simulink model "HighwayLaneChangeTestBench"  (R2024b)
settings: Solver=FixedStepAuto  StartTime=0.0  StopTime=scenario.StopTime  FixedStep=Ts  RelTol=1e-3
PostLoadFcn:
  | helperSLHighwayLaneChangeSetup;
values from neighbouring files (symbols this model uses):
  camera = cameraParams(egoActor)    [helperSLHighwayLaneChangeSetup.m]
undefined symbols (not defined in the file or in its folder): actorProfiles, driving, egoFrontExt, egoTTC, enableCCBehavior, enableLCBehavior, enableLCFBehavior, frontSafetyGap, latDevCost, mapInfo, matlabshared, maxAccel, maxCurvature, maxPlanningHorizon, maxYawRate, minVelocity, nextTTC, preferredLane, rearSafetyGap, replanRate, setSpeed, speedCost, targetFrontExt, timeCost, timeHorizon, timeResolution, Ts
libraries: drivingscenarioandsensors x8, canoelib x5, sensorinslib x1
CloseFcn:
  | helperSLHighwayLaneChangeCleanUp;
settings Model: Creator=The MathWorks, Inc.  LastModifiedBy=USER
settings SolverCC: ZeroCrossAlgorithm=Adaptive  AlgebraicLoopSolver=TrustRegion  MaxZcPerStep=1
settings DataIOCC: SaveOutput=off  ReturnWorkspaceOutputs=off
settings OptimizationCC: ReuseModelBlockBuffer=off
settings DebuggingCC: MaskedZcDiagnostic=none  IgnoredZcDiagnostic=none  UnconnectedInputMsg=warning  UnconnectedOutputMsg=warning  UnconnectedLineMsg=warning  BusObjectLabelMismatch=none  SubsystemReferenceDiagnosticForUnitTest=warning
settings ModelReferenceCC: EnableRefExpFcnMdlSchedulingChecks=on
settings RTWCC: GPUComputeCapability=3.5  DLArmComputeVersion=19.05

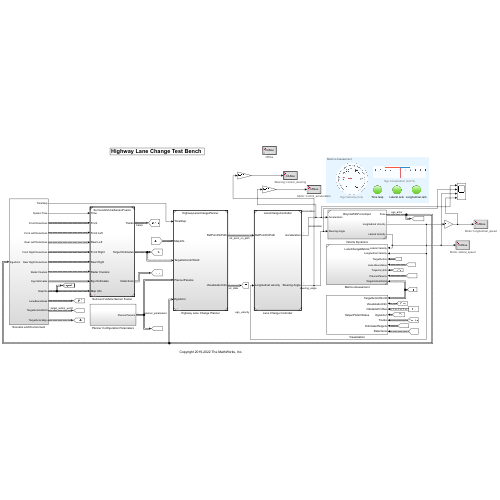
[thumbnail: Simulink's stored preview of the top-level diagram]
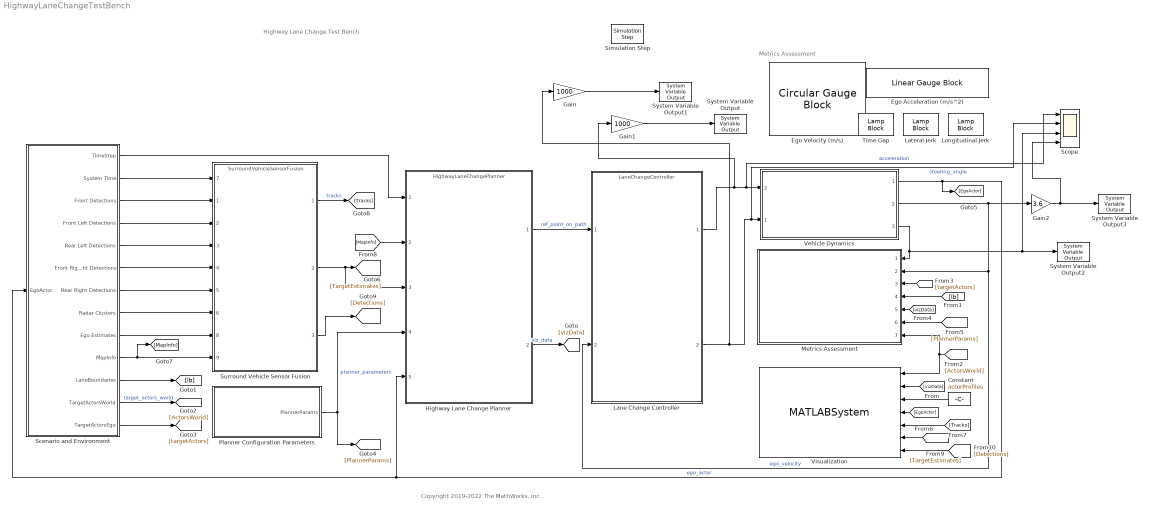
== system HighwayLaneChangeTestBench ==
  note: Copyright 2019-2022 The MathWorks, Inc.
  note: Metrics Assessment
  note: Highway Lane Change Test Bench
  Constant : Constant  Value=actorProfiles  OutDataTypeStr=Bus: BusActorProfiles
  Ego Acceleration (m/s^2) : LinearGaugeBlock  LabelPosition=Hide  ScaleMin=-5  ScaleMax=5
  Ego Velocity (m/s) : CircularGaugeBlock  LabelPosition=Hide  ScaleMax=50  TickInterval=5
  Gain : Gain  Gain=1000
  Gain1 : Gain  Gain=1000
  Gain2 : Gain  Gain=3.6
  Highway Lane Change Planner : ModelReference  ModelNameDialog=HighwayLaneChangePlanner.slx  SimulationMode=Normal  ModelReferenceVersion=10.0
  Lane Change Controller : ModelReference  ModelNameDialog=LaneChangeController.slx  SimulationMode=Normal  ModelReferenceVersion=9.0
  Lateral Jerk : LampBlock  LabelPosition=Hide
  Longitudinal Jerk : LampBlock  LabelPosition=Hide
  Metrics Assessment : Subsystem  ReferencedSubsystem=LaneChangeMetrics
  Planner Configuration Parameters : Subsystem
  Scenario and Environment : Subsystem
  Scope : Scope  NumInputPorts=4
  Simulation Step : canoelib/CANoe I//O/Simulation Step  mode=Offline
      settings: AttributesFormatString=%<mode>  SourceProductName=Vector CANoe
  Surround Vehicle Sensor Fusion : ModelReference  ModelNameDialog=SurroundVehicleSensorFusion.slx  SimulationMode=Normal  ModelReferenceVersion=10.0
      settings: PortSchema="{\"entries\":[{\"content\":{\"sides\":[{\"content\":{\"connectorIds\":[\"In7\",\"In1\",\"In2\",\"In3\",\"In4\",\"In5\",\"In6\",\"In8\",\"In9\"]},\"type\":\"ConnectorPlacement.EquallySpacedRectSide\",\"uuid\":\"babc32b8-473b-4a04-b824-251f7900e603\"},{\"content\":{\"connectorIds\":[\"Out1\",\"Out2\",\"Out3\"],\"side\":\"RIGHT\"},\"type\":\"ConnectorPlacement.EquallySpacedRectSide\",\"uuid\":\"6521796d-8396-47d7-a507-be3f8604ea95\"},{\"content\":{\"connectorIds\":[],\"side\":\"TOP\"},\"type\":\"ConnectorPlacement.EquallySpacedRectSide\",\"uuid\":\"3afcd3a1-01f6-437b-a186-b4f18cfd5e31\"}]},\"type\":\"ConnectorPlacement.EquallySpacedConnector\",\"uuid\":\"2716b65b-56e0-49c3-bc67-2edcf12b2a8e\"}],\"packageUris\":[\"http://schema.mathworks.com/mf0/Connector/R2020b\"],\"version\":\"1.0\"}"
  System Variable Output : canoelib/CANoe I//O/System Variable Output  nsName=Motor  sysVarName=control_acceleration  arrayIndex=-1  rawValue=Default  dataType=Default  dataTypeDB=double  hasEncoding=off  dataTypeCANoe=Get from CANoe
      settings: AttributesFormatString=%<nsName>::%<sysVarName>  SourceProductName=Vector CANoe
  System Variable Output1 : canoelib/CANoe I//O/System Variable Output  nsName=Steering  sysVarName=control_steering  arrayIndex=-1  rawValue=Default  dataType=Default  dataTypeDB=int32  hasEncoding=off  dataTypeCANoe=Get from CANoe
      settings: AttributesFormatString=%<nsName>::%<sysVarName>  SourceProductName=Vector CANoe
  System Variable Output2 : canoelib/CANoe I//O/System Variable Output  nsName=Motor  sysVarName=lateral_speed  arrayIndex=-1  rawValue=Default  dataType=Default  dataTypeDB=int32  hasEncoding=off  dataTypeCANoe=Get from CANoe
      settings: AttributesFormatString=%<nsName>::%<sysVarName>  SourceProductName=Vector CANoe
  System Variable Output3 : canoelib/CANoe I//O/System Variable Output  nsName=Motor  sysVarName=longitudinal_speed  arrayIndex=-1  rawValue=Default  dataType=Default  dataTypeDB=int32  hasEncoding=off  dataTypeCANoe=Get from CANoe
      settings: AttributesFormatString=%<nsName>::%<sysVarName>  SourceProductName=Vector CANoe
  Time Gap : LampBlock  LabelPosition=Hide
  Vehicle Dynamics : Subsystem  ReferencedSubsystem=BicycleWithForceInput
      settings: PortSchema="{\"entries\":[{\"content\":{\"sides\":[{\"content\":{\"connectorIds\":[\"In2\",\"In1\"]},\"type\":\"ConnectorPlacement.EquallySpacedRectSide\",\"uuid\":\"f63f66bc-f59a-4e63-885b-0681004bade6\"},{\"content\":{\"connectorIds\":[\"Out1\",\"Out2\",\"Out3\"],\"side\":\"RIGHT\"},\"type\":\"ConnectorPlacement.EquallySpacedRectSide\",\"uuid\":\"8ac8ea57-0210-4a13-ad95-4f0a9335ab33\"},{\"content\":{\"side\":\"TOP\"},\"type\":\"ConnectorPlacement.EquallySpacedRectSide\",\"uuid\":\"6d0b300d-41b2-47ad-8d2f-35db0d33cdc5\"}]},\"type\":\"ConnectorPlacement.EquallySpacedConnector\",\"uuid\":\"3215dd89-c688-4582-a904-15ea546ef61a\"}],\"packageUris\":[\"http://schema.mathworks.com/mf0/Connector/R2020b\"],\"version\":\"1.0\"}"
  Visualization : MATLABSystem  System=HelperPlotLCStatus  ActorsInfo=Tracks  EnableTopView=on  EnableTrajTopView=on  EnableTracksTopView=on  EnableChaseView=on  EnableTrajChase=on  EnableCaplistChaseView=on  EnableTracksChaseView=on
      mask Type: HelperPlotLCStatus
      mask Display:
      | disp('HelperPlotLCStatus');
      | port_label('input',1,'TargetActorsWorld');
      | port_label('input',2,'VisualizationInfo');
      | port_label('input',3,'ObstacleProfiles');
      | port_label('input',4,'EgoActor');
      | port_label('input',5,'Tracks');
      | port_label('input',6,'EstimatedTargets');
      | port_label('input',7,'Detections');
  wires:
  Planner Configuration Parameters/1(PlannerParams) -> Highway Lane Change Planner/4, [PlannerParams]  "planner_parameters"
  Highway Lane Change Planner/2 -> [vizData]  "viz_data"
  Scenario and Environment/11(LaneBoundaries) -> [lb]
  [lb] -> Metrics Assessment/4
  Highway Lane Change Planner/1 -> Lane Change Controller/1  "ref_point_on_path"
  [ActorsWorld] -> Metrics Assessment/7, Visualization/1
  Scenario and Environment/12(TargetActorsWorld) -> [ActorsWorld]  "target_actors_world"
  Scenario and Environment/13(TargetActorsEgo) -> [targetActors]
  [targetActors] -> Metrics Assessment/3
  Scenario and Environment/1(TimeStep) -> Highway Lane Change Planner/1
  Vehicle Dynamics/1 -> Scenario and Environment/1(EgoActor), Highway Lane Change Planner/5, [EgoActor]  "ego_actor"
  Vehicle Dynamics/2 -> Gain2/1, Lane Change Controller/2, Metrics Assessment/2  "ego_velocity"
  Lane Change Controller/2 -> Gain/1, Scope/2, Vehicle Dynamics/1  "steering_angle"
  Lane Change Controller/1 -> Gain1/1, Scope/1, Vehicle Dynamics/2  "acceleration"
  [vizData] -> Metrics Assessment/5
  [PlannerParams] -> Metrics Assessment/6
  Scenario and Environment/3(Front Detections) -> Surround Vehicle Sensor Fusion/1
  Scenario and Environment/4(Front Left Detections) -> Surround Vehicle Sensor Fusion/2
  Scenario and Environment/5(" Rear Left Detections") -> Surround Vehicle Sensor Fusion/3
  Scenario and Environment/6(Front Right Detections) -> Surround Vehicle Sensor Fusion/4
  Scenario and Environment/7(Rear Right Detections) -> Surround Vehicle Sensor Fusion/5
  Scenario and Environment/8(Radar Clusters) -> Surround Vehicle Sensor Fusion/6
  Scenario and Environment/9(Ego Estimates) -> Surround Vehicle Sensor Fusion/8
  [vizData] -> Visualization/2
  Constant/1 -> Visualization/3
  Scenario and Environment/10(MapInfo) -> [MapInfo], Surround Vehicle Sensor Fusion/9
  [MapInfo] -> Highway Lane Change Planner/2
  Surround Vehicle Sensor Fusion/2 -> Highway Lane Change Planner/3, [TargetEstimates]
  Surround Vehicle Sensor Fusion/1 -> [Tracks]  "tracks"
  Surround Vehicle Sensor Fusion/3 -> [Detections]
  [Tracks] -> Visualization/5
  [Detections] -> Visualization/7
  [EgoActor] -> Visualization/4
  [TargetEstimates] -> Visualization/6
  Scenario and Environment/2(System Time) -> Surround Vehicle Sensor Fusion/7
  Vehicle Dynamics/3 -> Metrics Assessment/1, System Variable Output2/1, Scope/3
  Gain/1 -> System Variable Output1/1
  Gain1/1 -> System Variable Output/1
  Gain2/1 -> Scope/4, System Variable Output3/1

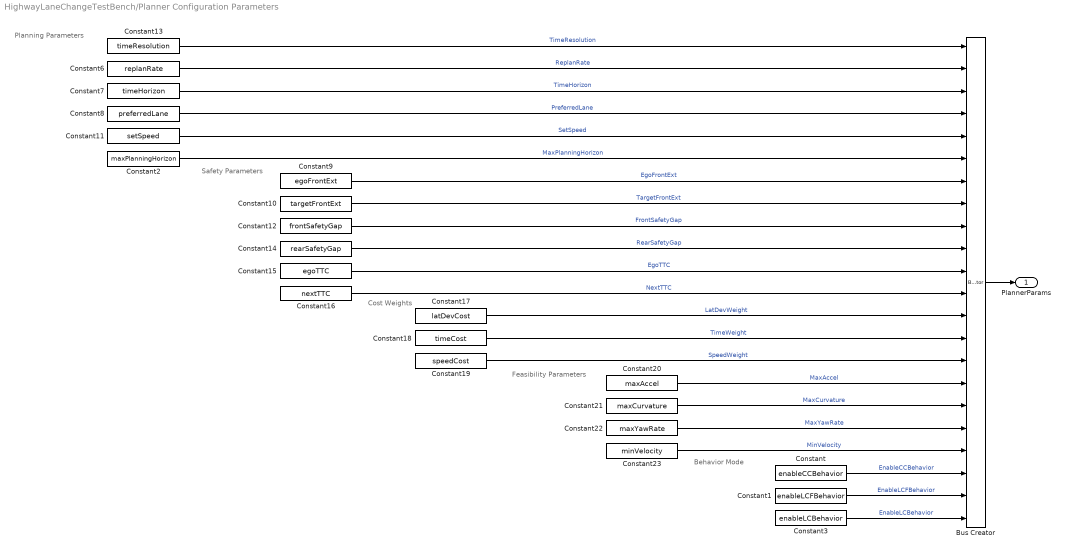
== system HighwayLaneChangeTestBench/Planner Configuration Parameters ==
  note: Planning Parameters
  note: Safety Parameters
  note: Cost Weights
  note: Feasibility Parameters
  note: Behavior Mode
  Bus Creator : BusCreator  Inputs=22  OutDataTypeStr=Bus: BusPlannerParams  NonVirtualBus=on
  Constant : Constant  Value=enableCCBehavior
  Constant1 : Constant  Value=enableLCFBehavior
  Constant10 : Constant  Value=targetFrontExt
  Constant11 : Constant  Value=setSpeed
  Constant12 : Constant  Value=frontSafetyGap
  Constant13 : Constant  Value=timeResolution
  Constant14 : Constant  Value=rearSafetyGap
  Constant15 : Constant  Value=egoTTC
  Constant16 : Constant  Value=nextTTC
  Constant17 : Constant  Value=latDevCost
  Constant18 : Constant  Value=timeCost
  Constant19 : Constant  Value=speedCost
  Constant2 : Constant  Value=maxPlanningHorizon
  Constant20 : Constant  Value=maxAccel
  Constant21 : Constant  Value=maxCurvature
  Constant22 : Constant  Value=maxYawRate
  Constant23 : Constant  Value=minVelocity
  Constant3 : Constant  Value=enableLCBehavior
  Constant6 : Constant  Value=replanRate
  Constant7 : Constant  Value=timeHorizon
  Constant8 : Constant  Value=preferredLane
  Constant9 : Constant  Value=egoFrontExt
  PlannerParams : Outport  OutDataTypeStr=Bus: BusPlannerParams
  wires:
  Constant19/1 -> Bus Creator/15  "SpeedWeight"
  Constant15/1 -> Bus Creator/11  "EgoTTC"
  Constant12/1 -> Bus Creator/9  "FrontSafetyGap"
  Constant6/1 -> Bus Creator/2  "ReplanRate"
  Constant14/1 -> Bus Creator/10  "RearSafetyGap"
  Constant20/1 -> Bus Creator/16  "MaxAccel"
  Constant18/1 -> Bus Creator/14  "TimeWeight"
  Constant11/1 -> Bus Creator/5  "SetSpeed"
  Constant13/1 -> Bus Creator/1  "TimeResolution"
  Constant23/1 -> Bus Creator/19  "MinVelocity"
  Constant9/1 -> Bus Creator/7  "EgoFrontExt"
  Constant16/1 -> Bus Creator/12  "NextTTC"
  Constant10/1 -> Bus Creator/8  "TargetFrontExt"
  Constant7/1 -> Bus Creator/3  "TimeHorizon"
  Constant21/1 -> Bus Creator/17  "MaxCurvature"
  Constant8/1 -> Bus Creator/4  "PreferredLane"
  Constant17/1 -> Bus Creator/13  "LatDevWeight"
  Bus Creator/1 -> PlannerParams/1
  Constant22/1 -> Bus Creator/18  "MaxYawRate"
  Constant/1 -> Bus Creator/20  "EnableCCBehavior"
  Constant1/1 -> Bus Creator/21  "EnableLCFBehavior"
  Constant3/1 -> Bus Creator/22  "EnableLCBehavior"
  Constant2/1 -> Bus Creator/6  "MaxPlanningHorizon"

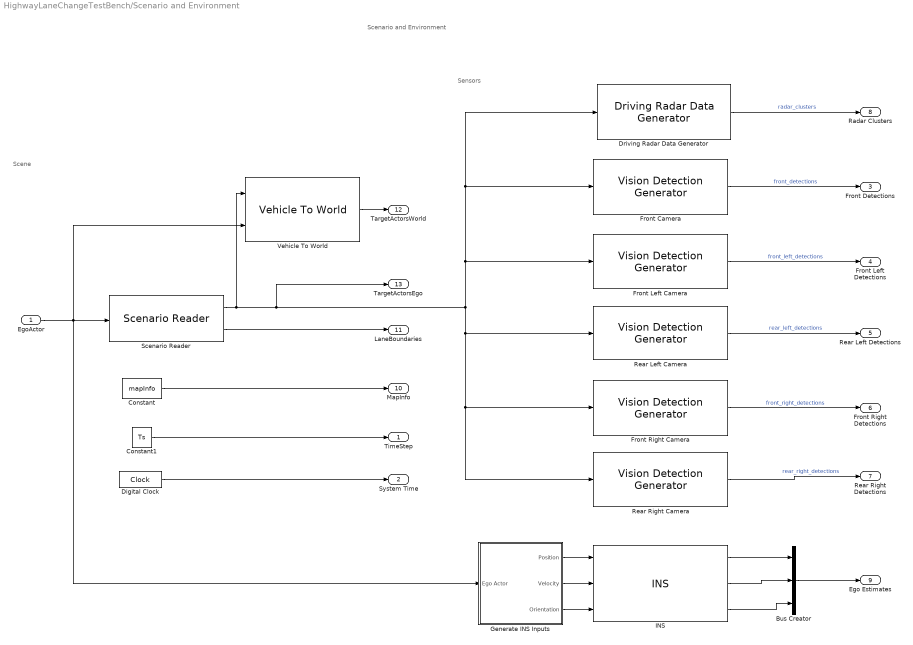
== system HighwayLaneChangeTestBench/Scenario and Environment ==
  note: Sensors
  note: Scene
  note: Scenario and Environment
  EgoActor : Inport
  Bus Creator : BusCreator  Inputs=3
  Constant : Constant  Value=mapInfo  OutDataTypeStr=Bus: BusMapInfo
  Constant1 : Constant  Value=Ts
  Digital Clock : DigitalClock  SampleTime=Ts
  Driving Radar Data Generator : drivingscenarioandsensors/Driving Radar Data Generator  SensorIndex=1  UpdateRate=10  MountingLocation=radar.Position  MountingAngles=radar.Rotation  HasElevation=off  HasRangeRate=on  HasNoise=on  HasFalseAlarms=off  HasOcclusion=off  MaxNumReportsSource=Property  MaxNumReports=50  TargetReportFormat=Clustered detections  DetectionCoordinates=Sensor spherical  TrackCoordinates=Body  BusNameSource=Property  BusName=BusDrivingRadarDataGenerator  SimulateUsing=Interpreted execution  AzimuthResolution=4  ElevationResolution=5  RangeResolution=2.5  RangeRateResolution=0.5  AzimuthBiasFraction=0.1  ElevationBiasFraction=0.1  RangeBiasFraction=0.05  RangeRateBiasFraction=0.05  FieldOfView=radar.FieldOfView  RangeLimits=radar.DetectionRanges  RangeRateLimits=[ -100, 100 ]  DetectionProbability=1  FalseAlarmRate=1e-06  ReferenceRange=100  ReferenceRCS=10  CenterFrequency=77e9  FilterInitializationFcn=initcvekf  ConfirmationThreshold=[2 3]  DeletionThreshold=[5 5]  InitialSeedSource=Repeatable  InitialSeed=0  UsedSeed=matlabshared.tracking.internal.SimulinkUtilities.seedManager(gcb)  ProfilesSource=From Scenario Reader block  ProfilesParameters=driving.internal.ActorProfilesRadarParameters  ProfilesExpression=struct('ClassID',0,'Length',4.7,'Width',1.8,'Height',1.4,'OriginOffset',[-1.35 0 0],'RCSPattern',[10 10;10 10],'RCSAzimuthAngles',[-180 180],'RCSElevationAngles',[-90 90])
  "Front Camera " : drivingscenarioandsensors/Vision Detection Generator  SensorIndex=2  DetectorOutput=Objects only  UpdateInterval=0.05  LaneUpdateInterval=0.1  SensorLocation=camera(1).Position(1:2)  Height=camera(1).Position(3)  Yaw=camera(1).Rotation(3)  Pitch=camera(1).Rotation(2)  Roll=camera(1).Rotation(1)  BusNameSource=Auto  BusName=BusObjectDetections  BusName2Source=Auto  BusName2=BusLaneDetections  MaxNumDetectionsSource=Property  MaxNumDetections=20  MaxNumLanesSource=Property  MaxNumLanes=30  DetectionCoordinates=Ego Cartesian  SimulateUsing=Interpreted execution  MaxRange=camera(1).DetectionRanges(2)  BoundingBoxAccuracy=1  ProcessNoiseIntensity=1  MaxSpeed=50  MaxAllowedOcclusion=0.99  MinObjectImageSize=[6 6]  DetectionProbability=0.95  FalsePositivesPerImage=0.02  MinLaneImageSize=[20 3]  LaneBoundaryAccuracy=3  HasNoise=off  InitialSeedSource=Specify seed  InitialSeed=0  UsedSeed=0  ActorProfilesSource=From Scenario Reader block  ActorProfilesParameters=driving.internal.ActorProfilesParameters  ActorProfilesExpression=[struct('ActorID',1,'ClassID',1,'Length',4.7,'Width',1.8,'Height',1.4,'OriginOffset',[-1.35 0 0],'MeshVertices',[3.7 -0.9 1.4;3.7 0.9 1.4;-1 0.9 1.4;-1 -0.9 1.4;3.7 -0.9 0;3.7 0.9 0;-1 0.9 0;-1 -0.9 0],'MeshFaces',[6 2 1;1 5 6;8 4 3;3 7 8;6 7 3;3 2 6;5 1 4;4 8 5;4 1 2;2 3 4;7 6 5;5 8 7],'RCSPattern',[10 10;10 10],'RCSAzimuthAngles',[-180 180],'RCSElevationAngles',[-90 90]); struct('ActorID',2,'ClassID',1,'Length',4.7,'Width',1.8,'Height',1.4,'OriginOffset',[-1.35 0 0],'MeshVertices',[3.7 -0.9 1.4;3.7 0.9 1.4;-1 0.9 1.4;-1 -0.9 1.4;3.7 -0.9 0;3.7 0.9 0;-1 0.9 0;-1 -0.9 0],'MeshFaces',[6 2 1;1 5 6;8 4 3;3 7 8;6 7 3;3 2 6;5 1 4;4 8 5;4 1 2;2 3 4;7 6 5;5 8 7],'RCSPattern',[10 10;10 10],'RCSAzimuthAngles',[-180 180],'RCSElevationAngles',[-90 90]); struct('ActorID',3,'ClassID',1,'Length',4.7,'Width',1.8,'Height',1.4,'OriginOffset',[-1.35 0 0],'MeshVertices',[3.7 -0.9 1.4;3.7 0.9 1.4;-1 0.9 1.4;-1 -0.9 1.4;3.7 -0.9 0;3.7 0.9 0;-1 0.9 0;-1 -0.9 0],'MeshFaces',[6 2 1;1 5 6;8 4 3;3 7 8;6 7 3;3 2 6;5 1 4;4 8 5;4 1 2;2 3 4;7 6 5;5 8 7],'RCSPattern',[10 10;10 10],'RCSAzimuthAngles',[-180 180],'RCSElevationAngles',[-90 90]); struct('ActorID',4,'ClassID',1,'Length',4.7,'Width',1.8,'Height',1.4,'OriginOffset',[-1.35 0 0],'MeshVertices',[3.7 -0.9 1.4;3.7 0.9 1.4;-1 0.9 1.4;-1 -0.9 1.4;3.7 -0.9 0;3.7 0.9 0;-1 0.9 0;-1 -0.9 0],'MeshFaces',[6 2 1;1 5 6;8 4 3;3 7 8;6 7 3;3 2 6;5 1 4;4 8 5;4 1 2;2 3 4;7 6 5;5 8 7],'RCSPattern',[10 10;10 10],'RCSAzimuthAngles',[-180 180],'RCSElevationAngles',[-90 90])]  Intrinsics=driving.internal.cameraIntrinsics('FocalLength',camera(1).FocalLength,'PrincipalPoint',camera(1).PrincipalPoint,'ImageSize',camera(1).ImageSize,'RadialDistortion',[0 0],'TangentialDistortion',[0 0],'Skew',0)
  Front Left Camera : drivingscenarioandsensors/Vision Detection Generator  SensorIndex=3  DetectorOutput=Objects only  UpdateInterval=0.05  LaneUpdateInterval=0.1  SensorLocation=camera(2).Position(1:2)  Height=camera(2).Position(3)  Yaw=camera(2).Rotation(3)  Pitch=camera(2).Rotation(2)  Roll=camera(2).Rotation(1)  BusNameSource=Auto  BusName=BusObjectDetections  BusName2Source=Auto  BusName2=BusLaneDetections  MaxNumDetectionsSource=Property  MaxNumDetections=20  MaxNumLanesSource=Property  MaxNumLanes=30  DetectionCoordinates=Ego Cartesian  SimulateUsing=Interpreted execution  MaxRange=camera(2).DetectionRanges(2)  BoundingBoxAccuracy=1  ProcessNoiseIntensity=1  MaxSpeed=50  MaxAllowedOcclusion=0.99  MinObjectImageSize=[6 6]  DetectionProbability=0.96  FalsePositivesPerImage=0.02  MinLaneImageSize=[20 3]  LaneBoundaryAccuracy=3  HasNoise=off  InitialSeedSource=Specify seed  InitialSeed=0.1  UsedSeed=0  ActorProfilesSource=From Scenario Reader block  ActorProfilesParameters=driving.internal.ActorProfilesParameters  ActorProfilesExpression=[struct('ActorID',1,'ClassID',1,'Length',4.7,'Width',1.8,'Height',1.4,'OriginOffset',[-1.35 0 0],'MeshVertices',[3.7 -0.9 1.4;3.7 0.9 1.4;-1 0.9 1.4;-1 -0.9 1.4;3.7 -0.9 0;3.7 0.9 0;-1 0.9 0;-1 -0.9 0],'MeshFaces',[6 2 1;1 5 6;8 4 3;3 7 8;6 7 3;3 2 6;5 1 4;4 8 5;4 1 2;2 3 4;7 6 5;5 8 7],'RCSPattern',[10 10;10 10],'RCSAzimuthAngles',[-180 180],'RCSElevationAngles',[-90 90]); struct('ActorID',2,'ClassID',1,'Length',4.7,'Width',1.8,'Height',1.4,'OriginOffset',[-1.35 0 0],'MeshVertices',[3.7 -0.9 1.4;3.7 0.9 1.4;-1 0.9 1.4;-1 -0.9 1.4;3.7 -0.9 0;3.7 0.9 0;-1 0.9 0;-1 -0.9 0],'MeshFaces',[6 2 1;1 5 6;8 4 3;3 7 8;6 7 3;3 2 6;5 1 4;4 8 5;4 1 2;2 3 4;7 6 5;5 8 7],'RCSPattern',[10 10;10 10],'RCSAzimuthAngles',[-180 180],'RCSElevationAngles',[-90 90]); struct('ActorID',3,'ClassID',1,'Length',4.7,'Width',1.8,'Height',1.4,'OriginOffset',[-1.35 0 0],'MeshVertices',[3.7 -0.9 1.4;3.7 0.9 1.4;-1 0.9 1.4;-1 -0.9 1.4;3.7 -0.9 0;3.7 0.9 0;-1 0.9 0;-1 -0.9 0],'MeshFaces',[6 2 1;1 5 6;8 4 3;3 7 8;6 7 3;3 2 6;5 1 4;4 8 5;4 1 2;2 3 4;7 6 5;5 8 7],'RCSPattern',[10 10;10 10],'RCSAzimuthAngles',[-180 180],'RCSElevationAngles',[-90 90]); struct('ActorID',4,'ClassID',1,'Length',4.7,'Width',1.8,'Height',1.4,'OriginOffset',[-1.35 0 0],'MeshVertices',[3.7 -0.9 1.4;3.7 0.9 1.4;-1 0.9 1.4;-1 -0.9 1.4;3.7 -0.9 0;3.7 0.9 0;-1 0.9 0;-1 -0.9 0],'MeshFaces',[6 2 1;1 5 6;8 4 3;3 7 8;6 7 3;3 2 6;5 1 4;4 8 5;4 1 2;2 3 4;7 6 5;5 8 7],'RCSPattern',[10 10;10 10],'RCSAzimuthAngles',[-180 180],'RCSElevationAngles',[-90 90])]  Intrinsics=driving.internal.cameraIntrinsics('FocalLength',camera(2).FocalLength,'PrincipalPoint',camera(2).PrincipalPoint,'ImageSize',camera(2).ImageSize,'RadialDistortion',[0 0],'TangentialDistortion',[0 0],'Skew',0)
  Front Right Camera : drivingscenarioandsensors/Vision Detection Generator  SensorIndex=5  DetectorOutput=Objects only  UpdateInterval=0.05  LaneUpdateInterval=0.1  SensorLocation=camera(4).Position(1:2)  Height=camera(4).Position(3)  Yaw=camera(4).Rotation(3)  Pitch=camera(4).Rotation(2)  Roll=camera(4).Rotation(1)  BusNameSource=Auto  BusName=BusObjectDetections  BusName2Source=Auto  BusName2=BusLaneDetections  MaxNumDetectionsSource=Property  MaxNumDetections=20  MaxNumLanesSource=Property  MaxNumLanes=30  DetectionCoordinates=Ego Cartesian  SimulateUsing=Interpreted execution  MaxRange=camera(4).DetectionRanges(2)  BoundingBoxAccuracy=1  ProcessNoiseIntensity=1  MaxSpeed=50  MaxAllowedOcclusion=0.99  MinObjectImageSize=[6 6]  DetectionProbability=0.96  FalsePositivesPerImage=0.02  MinLaneImageSize=[20 3]  LaneBoundaryAccuracy=3  HasNoise=off  InitialSeedSource=Specify seed  InitialSeed=0.3  UsedSeed=0  ActorProfilesSource=From Scenario Reader block  ActorProfilesParameters=driving.internal.ActorProfilesParameters  ActorProfilesExpression=[struct('ActorID',1,'ClassID',1,'Length',4.7,'Width',1.8,'Height',1.4,'OriginOffset',[-1.35 0 0],'MeshVertices',[3.7 -0.9 1.4;3.7 0.9 1.4;-1 0.9 1.4;-1 -0.9 1.4;3.7 -0.9 0;3.7 0.9 0;-1 0.9 0;-1 -0.9 0],'MeshFaces',[6 2 1;1 5 6;8 4 3;3 7 8;6 7 3;3 2 6;5 1 4;4 8 5;4 1 2;2 3 4;7 6 5;5 8 7],'RCSPattern',[10 10;10 10],'RCSAzimuthAngles',[-180 180],'RCSElevationAngles',[-90 90]); struct('ActorID',2,'ClassID',1,'Length',4.7,'Width',1.8,'Height',1.4,'OriginOffset',[-1.35 0 0],'MeshVertices',[3.7 -0.9 1.4;3.7 0.9 1.4;-1 0.9 1.4;-1 -0.9 1.4;3.7 -0.9 0;3.7 0.9 0;-1 0.9 0;-1 -0.9 0],'MeshFaces',[6 2 1;1 5 6;8 4 3;3 7 8;6 7 3;3 2 6;5 1 4;4 8 5;4 1 2;2 3 4;7 6 5;5 8 7],'RCSPattern',[10 10;10 10],'RCSAzimuthAngles',[-180 180],'RCSElevationAngles',[-90 90]); struct('ActorID',3,'ClassID',1,'Length',4.7,'Width',1.8,'Height',1.4,'OriginOffset',[-1.35 0 0],'MeshVertices',[3.7 -0.9 1.4;3.7 0.9 1.4;-1 0.9 1.4;-1 -0.9 1.4;3.7 -0.9 0;3.7 0.9 0;-1 0.9 0;-1 -0.9 0],'MeshFaces',[6 2 1;1 5 6;8 4 3;3 7 8;6 7 3;3 2 6;5 1 4;4 8 5;4 1 2;2 3 4;7 6 5;5 8 7],'RCSPattern',[10 10;10 10],'RCSAzimuthAngles',[-180 180],'RCSElevationAngles',[-90 90]); struct('ActorID',4,'ClassID',1,'Length',4.7,'Width',1.8,'Height',1.4,'OriginOffset',[-1.35 0 0],'MeshVertices',[3.7 -0.9 1.4;3.7 0.9 1.4;-1 0.9 1.4;-1 -0.9 1.4;3.7 -0.9 0;3.7 0.9 0;-1 0.9 0;-1 -0.9 0],'MeshFaces',[6 2 1;1 5 6;8 4 3;3 7 8;6 7 3;3 2 6;5 1 4;4 8 5;4 1 2;2 3 4;7 6 5;5 8 7],'RCSPattern',[10 10;10 10],'RCSAzimuthAngles',[-180 180],'RCSElevationAngles',[-90 90])]  Intrinsics=driving.internal.cameraIntrinsics('FocalLength',camera(4).FocalLength,'PrincipalPoint',camera(4).PrincipalPoint,'ImageSize',camera(4).ImageSize,'RadialDistortion',[0 0],'TangentialDistortion',[0 0],'Skew',0)
  Generate INS Inputs : Subsystem  TreatAsAtomicUnit=on
  INS : sensorinslib/INS  MountingLocation=[0 0 0]  RollAccuracy=0.1  PitchAccuracy=0.1  YawAccuracy=0.1  PositionAccuracy=0.1  VelocityAccuracy=0.1  UseAccelAndAngVel=off  AccelerationAccuracy=0  AngularVelocityAccuracy=0  TimeInput=off  PositionErrorFactor=[0 0 0]  SeedDouble=67  SimulateUsing=Interpreted execution
  Rear Left Camera : drivingscenarioandsensors/Vision Detection Generator  SensorIndex=4  DetectorOutput=Objects only  UpdateInterval=0.05  LaneUpdateInterval=0.1  SensorLocation=camera(3).Position(1:2)  Height=camera(3).Position(3)  Yaw=camera(3).Rotation(3)  Pitch=camera(3).Rotation(2)  Roll=camera(3).Rotation(1)  BusNameSource=Auto  BusName=BusObjectDetections  BusName2Source=Auto  BusName2=BusLaneDetections  MaxNumDetectionsSource=Property  MaxNumDetections=20  MaxNumLanesSource=Property  MaxNumLanes=30  DetectionCoordinates=Ego Cartesian  SimulateUsing=Interpreted execution  MaxRange=camera(3).DetectionRanges(2)  BoundingBoxAccuracy=1  ProcessNoiseIntensity=1  MaxSpeed=50  MaxAllowedOcclusion=0.99  MinObjectImageSize=[6 6]  DetectionProbability=0.95  FalsePositivesPerImage=0.02  MinLaneImageSize=[20 3]  LaneBoundaryAccuracy=3  HasNoise=off  InitialSeedSource=Specify seed  InitialSeed=0.2  UsedSeed=0  ActorProfilesSource=From Scenario Reader block  ActorProfilesParameters=driving.internal.ActorProfilesParameters  ActorProfilesExpression=[struct('ActorID',1,'ClassID',1,'Length',4.7,'Width',1.8,'Height',1.4,'OriginOffset',[-1.35 0 0],'MeshVertices',[3.7 -0.9 1.4;3.7 0.9 1.4;-1 0.9 1.4;-1 -0.9 1.4;3.7 -0.9 0;3.7 0.9 0;-1 0.9 0;-1 -0.9 0],'MeshFaces',[6 2 1;1 5 6;8 4 3;3 7 8;6 7 3;3 2 6;5 1 4;4 8 5;4 1 2;2 3 4;7 6 5;5 8 7],'RCSPattern',[10 10;10 10],'RCSAzimuthAngles',[-180 180],'RCSElevationAngles',[-90 90]); struct('ActorID',2,'ClassID',1,'Length',4.7,'Width',1.8,'Height',1.4,'OriginOffset',[-1.35 0 0],'MeshVertices',[3.7 -0.9 1.4;3.7 0.9 1.4;-1 0.9 1.4;-1 -0.9 1.4;3.7 -0.9 0;3.7 0.9 0;-1 0.9 0;-1 -0.9 0],'MeshFaces',[6 2 1;1 5 6;8 4 3;3 7 8;6 7 3;3 2 6;5 1 4;4 8 5;4 1 2;2 3 4;7 6 5;5 8 7],'RCSPattern',[10 10;10 10],'RCSAzimuthAngles',[-180 180],'RCSElevationAngles',[-90 90]); struct('ActorID',3,'ClassID',1,'Length',4.7,'Width',1.8,'Height',1.4,'OriginOffset',[-1.35 0 0],'MeshVertices',[3.7 -0.9 1.4;3.7 0.9 1.4;-1 0.9 1.4;-1 -0.9 1.4;3.7 -0.9 0;3.7 0.9 0;-1 0.9 0;-1 -0.9 0],'MeshFaces',[6 2 1;1 5 6;8 4 3;3 7 8;6 7 3;3 2 6;5 1 4;4 8 5;4 1 2;2 3 4;7 6 5;5 8 7],'RCSPattern',[10 10;10 10],'RCSAzimuthAngles',[-180 180],'RCSElevationAngles',[-90 90]); struct('ActorID',4,'ClassID',1,'Length',4.7,'Width',1.8,'Height',1.4,'OriginOffset',[-1.35 0 0],'MeshVertices',[3.7 -0.9 1.4;3.7 0.9 1.4;-1 0.9 1.4;-1 -0.9 1.4;3.7 -0.9 0;3.7 0.9 0;-1 0.9 0;-1 -0.9 0],'MeshFaces',[6 2 1;1 5 6;8 4 3;3 7 8;6 7 3;3 2 6;5 1 4;4 8 5;4 1 2;2 3 4;7 6 5;5 8 7],'RCSPattern',[10 10;10 10],'RCSAzimuthAngles',[-180 180],'RCSElevationAngles',[-90 90])]  Intrinsics=driving.internal.cameraIntrinsics('FocalLength',camera(3).FocalLength,'PrincipalPoint',camera(3).PrincipalPoint,'ImageSize',camera(3).ImageSize,'RadialDistortion',[0 0],'TangentialDistortion',[0 0],'Skew',0)
  Rear Right Camera : drivingscenarioandsensors/Vision Detection Generator  SensorIndex=6  DetectorOutput=Objects only  UpdateInterval=0.05  LaneUpdateInterval=0.1  SensorLocation=camera(5).Position(1:2)  Height=camera(5).Position(3)  Yaw=camera(5).Rotation(3)  Pitch=camera(5).Rotation(2)  Roll=camera(5).Rotation(1)  BusNameSource=Auto  BusName=BusObjectDetections  BusName2Source=Auto  BusName2=BusLaneDetections  MaxNumDetectionsSource=Property  MaxNumDetections=20  MaxNumLanesSource=Property  MaxNumLanes=30  DetectionCoordinates=Ego Cartesian  SimulateUsing=Interpreted execution  MaxRange=camera(5).DetectionRanges(2)  BoundingBoxAccuracy=1  ProcessNoiseIntensity=1  MaxSpeed=50  MaxAllowedOcclusion=0.99  MinObjectImageSize=[6 6]  DetectionProbability=0.95  FalsePositivesPerImage=0.02  MinLaneImageSize=[20 3]  LaneBoundaryAccuracy=3  HasNoise=off  InitialSeedSource=Specify seed  InitialSeed=0.4  UsedSeed=0  ActorProfilesSource=From Scenario Reader block  ActorProfilesParameters=driving.internal.ActorProfilesParameters  ActorProfilesExpression=[struct('ActorID',1,'ClassID',1,'Length',4.7,'Width',1.8,'Height',1.4,'OriginOffset',[-1.35 0 0],'MeshVertices',[3.7 -0.9 1.4;3.7 0.9 1.4;-1 0.9 1.4;-1 -0.9 1.4;3.7 -0.9 0;3.7 0.9 0;-1 0.9 0;-1 -0.9 0],'MeshFaces',[6 2 1;1 5 6;8 4 3;3 7 8;6 7 3;3 2 6;5 1 4;4 8 5;4 1 2;2 3 4;7 6 5;5 8 7],'RCSPattern',[10 10;10 10],'RCSAzimuthAngles',[-180 180],'RCSElevationAngles',[-90 90]); struct('ActorID',2,'ClassID',1,'Length',4.7,'Width',1.8,'Height',1.4,'OriginOffset',[-1.35 0 0],'MeshVertices',[3.7 -0.9 1.4;3.7 0.9 1.4;-1 0.9 1.4;-1 -0.9 1.4;3.7 -0.9 0;3.7 0.9 0;-1 0.9 0;-1 -0.9 0],'MeshFaces',[6 2 1;1 5 6;8 4 3;3 7 8;6 7 3;3 2 6;5 1 4;4 8 5;4 1 2;2 3 4;7 6 5;5 8 7],'RCSPattern',[10 10;10 10],'RCSAzimuthAngles',[-180 180],'RCSElevationAngles',[-90 90]); struct('ActorID',3,'ClassID',1,'Length',4.7,'Width',1.8,'Height',1.4,'OriginOffset',[-1.35 0 0],'MeshVertices',[3.7 -0.9 1.4;3.7 0.9 1.4;-1 0.9 1.4;-1 -0.9 1.4;3.7 -0.9 0;3.7 0.9 0;-1 0.9 0;-1 -0.9 0],'MeshFaces',[6 2 1;1 5 6;8 4 3;3 7 8;6 7 3;3 2 6;5 1 4;4 8 5;4 1 2;2 3 4;7 6 5;5 8 7],'RCSPattern',[10 10;10 10],'RCSAzimuthAngles',[-180 180],'RCSElevationAngles',[-90 90]); struct('ActorID',4,'ClassID',1,'Length',4.7,'Width',1.8,'Height',1.4,'OriginOffset',[-1.35 0 0],'MeshVertices',[3.7 -0.9 1.4;3.7 0.9 1.4;-1 0.9 1.4;-1 -0.9 1.4;3.7 -0.9 0;3.7 0.9 0;-1 0.9 0;-1 -0.9 0],'MeshFaces',[6 2 1;1 5 6;8 4 3;3 7 8;6 7 3;3 2 6;5 1 4;4 8 5;4 1 2;2 3 4;7 6 5;5 8 7],'RCSPattern',[10 10;10 10],'RCSAzimuthAngles',[-180 180],'RCSElevationAngles',[-90 90])]  Intrinsics=driving.internal.cameraIntrinsics('FocalLength',camera(5).FocalLength,'PrincipalPoint',camera(5).PrincipalPoint,'ImageSize',camera(5).ImageSize,'RadialDistortion',[0 0],'TangentialDistortion',[0 0],'Skew',0)
  Scenario Reader : drivingscenarioandsensors/Scenario Reader  ScenarioSource=From workspace  ScenarioFileName=CurevedRoadNetwork.mat  ScenarioVariableName=scenario  OutputCoordinateSystem=Vehicle coordinates  EgoVehicleSource=Input port  EgoVehicleActorID=egoInitialPose.ActorID  OrientVehiclesOnRoad=off  OutputEgoVehiclePose=off  OutputEgoVehicleState=off  SampleTime=0.1  LaneBoundaryOutput=Ego vehicle lane boundaries  LaneBoundaryDistance=0:0.5:60  LaneBoundaryLocation=Center of lane markings  BusNameSource=Property  BusName=BusActorsTruth  BusNumActorsSource=Scenario  BusNumActors=100  BusName2Source=Auto  BusName2=BusLaneBoundaries  BusNumLaneBoundariesSource=Scenario  BusNumLaneBoundaries=10  BusName3Source=Auto  BusName3=BusEgoActor  BusName4Source=Auto  BusName4=BusEgoState  ShowCoordinateLabels=on  SimulateUsing=Interpreted execution
  Vehicle To World : drivingscenarioandsensors/Vehicle To World  BusNameSource=Auto  BusName=BusVehicleToWorldActors  SimulateUsing=Interpreted execution
  TimeStep : Outport
  System Time : Outport  Port=2
  Front Detections : Outport  Port=3
  Front Left Detections : Outport  Port=4
  " Rear Left Detections" : Outport  Port=5
  Front Right Detections : Outport  Port=6
  Rear Right Detections : Outport  Port=7
  Radar Clusters : Outport  Port=8  OutDataTypeStr=Bus: BusDrivingRadarDataGenerator
  Ego Estimates : Outport  Port=9  OutDataTypeStr=Bus: BusEgoPose
  MapInfo : Outport  Port=10  OutDataTypeStr=Bus: BusMapInfo
  LaneBoundaries : Outport  Port=11
  TargetActorsWorld : Outport  Port=12  OutDataTypeStr=Bus: BusActorsTruth
  TargetActorsEgo : Outport  Port=13  OutDataTypeStr=Bus: BusActorsTruth
  wires:
  Scenario Reader/1 -> Driving Radar Data Generator/1, "Front Camera "/1, Front Left Camera/1, Rear Right Camera/1, Front Right Camera/1, Rear Left Camera/1, TargetActorsEgo/1, Vehicle To World/1
  Constant/1 -> MapInfo/1
  Constant1/1 -> TimeStep/1
  Rear Right Camera/1 -> Rear Right Detections/1  "rear_right_detections"
  Front Left Camera/1 -> Front Left Detections/1  "front_left_detections"
  Driving Radar Data Generator/1 -> Radar Clusters/1  "radar_clusters"
  Front Right Camera/1 -> Front Right Detections/1  "front_right_detections"
  Rear Left Camera/1 -> " Rear Left Detections"/1  "rear_left_detections"
  "Front Camera "/1 -> Front Detections/1  "front_detections"
  Scenario Reader/2 -> LaneBoundaries/1
  Vehicle To World/1 -> TargetActorsWorld/1
  INS/1 -> Bus Creator/1
  INS/3 -> Bus Creator/3
  EgoActor/1 -> Generate INS Inputs/1(Ego Actor), Vehicle To World/2, Scenario Reader/1
  Bus Creator/1 -> Ego Estimates/1
  INS/2 -> Bus Creator/2
  Generate INS Inputs/3(Orientation) -> INS/3
  Generate INS Inputs/2(Velocity) -> INS/2
  Generate INS Inputs/1(Position) -> INS/1
  Digital Clock/1 -> System Time/1

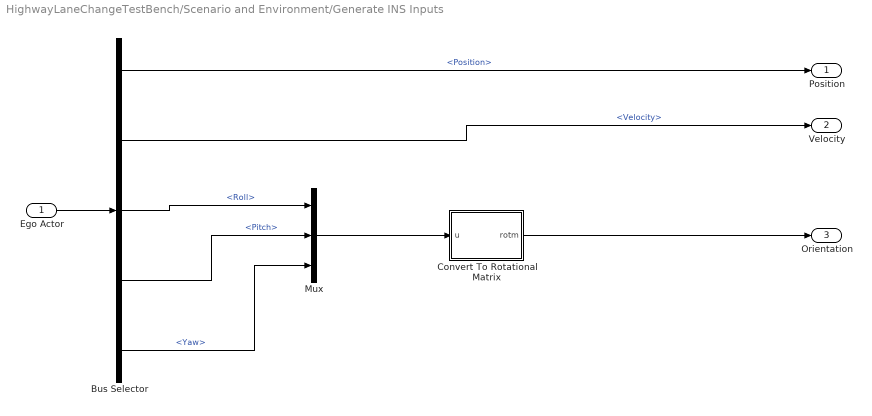
== system HighwayLaneChangeTestBench/Scenario and Environment/Generate INS Inputs ==
  Ego Actor : Inport
  Bus Selector : BusSelector  OutputSignals=Position,Velocity,Roll,Pitch,Yaw
  Convert To Rotational Matrix : MATLAB Function  TreatAsAtomicUnit=on
  Mux : Mux  Inputs=3
  Position : Outport
  Velocity : Outport  Port=2
  Orientation : Outport  Port=3
  wires:
  Bus Selector/2 -> Velocity/1  "<Velocity>"
  Bus Selector/1 -> Position/1  "<Position>"
  Bus Selector/5 -> Mux/3  "<Yaw>"
  Bus Selector/4 -> Mux/2  "<Pitch>"
  Bus Selector/3 -> Mux/1  "<Roll>"
  Ego Actor/1 -> Bus Selector/1
  Mux/1 -> Convert To Rotational Matrix/1(u)
  Convert To Rotational Matrix/1(rotm) -> Orientation/1

== matlab function HighwayLaneChangeTestBench/Scenario and Environment/Generate INS Inputs/Convert To Rotational Matrix ==
  data: u input; rotm output size=[3 3]
function rotm = eul2rotMatrix(u)
eul = u/180*pi;
rotm = eul2rotm(eul',"XYZ");
end
